simulink model "SistemaCompleto_PMSM"  (R2025a)
settings: Solver=VariableStepAuto  StartTime=0.0  StopTime=3  RelTol=1e-3
PostLoadFcn:
  | parametros_sistema_completo
  | run("parametros_sistema_completo.mlx")
values from neighbouring files (symbols this model uses):
  a_cu = 3.9e-3    (= 0.0039)    [parametros_sistema_completo.m]    (also in workspace_params.mat)
  b_eq = params.b_total    [calcular_matriz_AO.m]    (also in calculo_incertidumbre_y_control.m = b_m + b_l/(r^2); parametros_sistema_completo.m = 2.19444444444e-05; workspace_params.mat = 2.19444444444e-05)
  C_ts = C_ts * (1 + tol_pct)    [calculo_incertidumbre_y_control.m]    (also in parametros_sistema_completo.m = 0.818; workspace_params.mat = 0.818)
  g = 9.80665    [parametros_sistema_completo.m]    (also in workspace_params.mat)
  J_eq = params.J_total    [calcular_matriz_AO.m]    (also in calculo_incertidumbre_y_control.m = J_m + J_l/r^2; parametros_sistema_completo.m = 1.97847222222e-05; workspace_params.mat = 3.28055555556e-05)
  k_l = m*l_cm + m_l*l_l    [calculo_incertidumbre_y_control.m]    (also in parametros_sistema_completo.m = 0.25; workspace_params.mat = 0.625)
  L_d = L_d    * (1 - tol_pct)    [calculo_incertidumbre_y_control.m]    (also in parametros_sistema_completo.m = 0.0066; workspace_params.mat = 0.0066)
  L_ls = L_ls   * (1 - tol_pct)    [calculo_incertidumbre_y_control.m]    (also in parametros_sistema_completo.m = 0.0008; workspace_params.mat = 0.0008)
  L_q = L_q    * (1 - tol_pct)    [calculo_incertidumbre_y_control.m]    (also in parametros_sistema_completo.m = 0.0058; workspace_params.mat = 0.0058)
  lambda_r = lambda_r * (1 + tol_pct)    [calculo_incertidumbre_y_control.m]    (also in parametros_sistema_completo.m = 0.016; workspace_params.mat = 0.016)
  P_p = 3    [parametros_sistema_completo.m]    (also in workspace_params.mat)
  r = params.r_red    [calcular_matriz_AO.m]    (also in parametros_sistema_completo.m = 120; workspace_params.mat = 120)
  R_sREF = R_sREF * (1 - tol_pct)    [calculo_incertidumbre_y_control.m]    (also in parametros_sistema_completo.m = 1.02; workspace_params.mat = 1.02)
  R_ts_amb = R_ts_amb * (1 - tol_pct)    [calculo_incertidumbre_y_control.m]    (also in parametros_sistema_completo.m = 146.7; workspace_params.mat = 146.7)
  T_amb = 20    [parametros_sistema_completo.m]    (also in workspace_params.mat)
  T_sREF = 20    [parametros_sistema_completo.m]    (also in workspace_params.mat)
undefined symbols (not defined in the file or in its folder): i_ds_inicial
libraries: eeStairGenerator x2
settings Model: Creator=Francisco  LastModifiedBy=Francisco
settings DebuggingCC: UnderspecifiedInitializationDetection=Classic  MergeDetectMultiDrivingBlocksExec=none
settings ModelReferenceCC: PropagateSignalLabelsOutOfModel=off
settings RTWCC: GPUComputeCapability=3.5

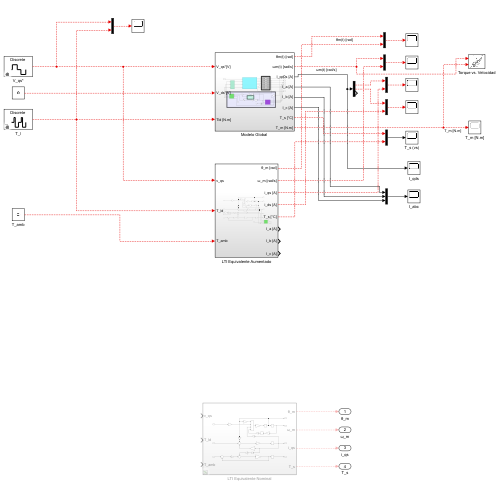
[thumbnail: Simulink's stored preview of the top-level diagram]
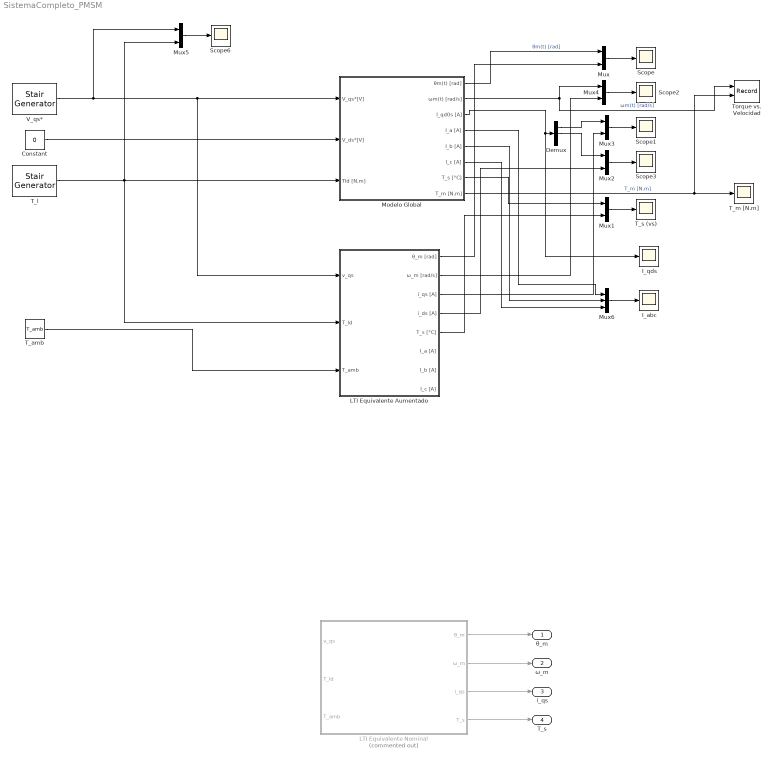
== system SistemaCompleto_PMSM ==
  Constant : Constant  Value=0
  Demux : Demux  Outputs=3
  I_abc : Scope
      settings: ActiveDisplayYMinimum=-11.027390626424687  ActiveDisplayYMaximum=9.9575916434176612  DataLoggingVariableName=ScopeData8
  I_qds : Scope
      settings: ActiveDisplayYMinimum=-9.49860290767503  ActiveDisplayYMaximum=9.6412352540190742  DataLoggingVariableName=ScopeData3
  LTI Equivalente Aumentado : Subsystem
  LTI Equivalente Nominal : Subsystem  Commented=on
  "Modelo Global " : Subsystem
  Mux{,1..5} (6 alike) : Mux  Inputs=2
  Mux6 : Mux  Inputs=3
  Scope{,1..3,6} (5 alike) : Scope
      Scope settings: ActiveDisplayYMinimum=-1  ActiveDisplayYMaximum=1
      Scope1 settings: ActiveDisplayYMinimum=-1  ActiveDisplayYMaximum=1  DataLoggingVariableName=ScopeData2
      Scope2 settings: ActiveDisplayYMinimum=-1  ActiveDisplayYMaximum=1
      Scope3 settings: ActiveDisplayYMinimum=-6.8361156933848816E-13  ActiveDisplayYMaximum=1.2107764476761756E-12  DataLoggingVariableName=ScopeData4
      Scope6 settings: ActiveDisplayYMinimum=-1  ActiveDisplayYMaximum=1  DataLoggingVariableName=ScopeData7
  T_amb : Constant  Value=T_amb
  T_l : eeStairGenerator/Stair Generator  LabelModeActiveChoice=Discrete  TimeInput=[0 0.3 0.5 0.9 1.3 1.5 1.9]  AmplitudeInput=[0 6.28 -6.28 0 6.28 -6.28 0]  SampleTime=0.001  RepeatPattern=off  OutDataTypeStr=double
      settings: LibrarySourceBlock=ee_sl_lib/General Control/Stair Generator
  T_m [N.m] : Scope
      settings: ActiveDisplayYMinimum=-0.86646302297159927  ActiveDisplayYMaximum=1.6077968765433432  DataLoggingVariableName=ScopeData6
  T_s (vs) : Scope
      settings: ActiveDisplayYMinimum=18.3730242701774  ActiveDisplayYMaximum=30.348736241613476  DataLoggingVariableName=ScopeData5
  Torque vs. Velocidad : Record  NumPorts=2.0  FileSettingsInternal="{\"entries\":[{\"content\":{\"excelSettings\":{\"content\":{},\"type\":\"Streamout.ExcelSettings\"},\"parquetSettings\":{\"content\":{},\"type\":\"Streamout.ParquetSettings\"}},\"type\":\"Streamout.FileSettingStorage\",\"uuid\":\"\"}],\"packageUris\":[\"http:\\/\\/schema.mathworks.com\\/mf0\\/streamout_blocks\\/R2020a\"],\"version\":\"1.0\"}"  FrameSettings=[0, 0]  Layout=[1 1]  SignalsInternal="{\"entries\":[{\"content\":{\"signals\":[{\"content\":{\"blockPath\":[],\"dimensions\":[1],\"domain\":\"\",\"lineColor\":\"#a2142f\",\"plots\":[ 1 ],\"port\":1,\"sid\":[\"\"],\"signalID\":1,\"signalName\":\"Modelo Global :2\"},\"type\":\"RecordBlkView.Signal\",\"uuid\":\"\"},{\"content\":{\"blockPath\":[],\"dimensions\":[1],\"domain\":\"\",\"lineColor\":\"#139fff\",\"plots\":[ 1 ],\"port\":2,\"sid\":[\"\"],\"signalID\":2,\"signalName\":\"Modelo Global :8\"},\"type\":\"RecordBlkView.Signal\",\"uuid\":\"\"},{\"content\":{\"blockPath\":[],\"dimensions\":[1],\"domain\":\"\",\"lineColor\":\"#77ac30\",\"lineWidth\":2,\"port\":1,\"sid\":[\"\"],\"signalID\":3},\"type\":\"RecordBlkView.Signal\",\"uuid\":\"\"},{\"content\":{\"blockPath\":[],\"dimensions\":[1],\"domain\":\"\",\"lineColor\":\"#4dbeee\",\"lineWidth\":2,\"port\":1,\"sid\":[\"\"],\"signalID\":4},\"type\":\"RecordBlkView.Signal\",\"uuid\":\"\"},{\"content\":{\"blockPath\":[],\"dimensions\":[1],\"domain\":\"\",\"lineColor\":\"#a2142f\",\"lineWidth\":2,\"port\":1,\"sid\":[\"\"],\"signalID\":5},\"type\":\"RecordBlkView.Signal\",\"uuid\":\"\"},{\"content\":{\"blockPath\":[],\"dimensions\":[1],\"domain\":\"\",\"lineColor\":\"#139fff\",\"lineWidth\":2,\"port\":1,\"sid\":[\"\"],\"signalID\":6},\"type\":\"RecordBlkView.Signal\",\"uuid\":\"\"}]},\"type\":\"RecordBlkView.InputSignals\",\"uuid\":\"\"}],\"packageUris\":[\"http:\\/\\/schema.mathworks.com\\/mf0\\/streamout_blocks\\/R2020a\"],\"version\":\"1.0\"}"  VisualizationBindings="{\"xyplotplugin\":{\"info\":[{\"series\":[{\"bindingParametersList\":[{\"parameter\":\"X-Axis\",\"signalID\":1,\"signalName\":\"Modelo Global :2\"},{\"parameter\":\"Y-Axis\",\"signalID\":2,\"signalName\":\"Modelo Global :8\"}],\"seriesID\":0}],\"subplotID\":1}]}}"  CompatibilityTag=XY
  V_qs* : eeStairGenerator/Stair Generator  LabelModeActiveChoice=Discrete  TimeInput=[0 0.1 0.7 1.1 1.7]  AmplitudeInput=[0 19.596 0 -19.596 0]  SampleTime=0.001  RepeatPattern=off  OutDataTypeStr=double
      settings: LibrarySourceBlock=ee_sl_lib/General Control/Stair Generator
  θ_m : Outport
  ω_m : Outport  Port=2
  i_qs : Outport  Port=3
  T_s : Outport  Port=4
  wires:
  LTI Equivalente Nominal/1(θ_m) -> θ_m/1
  LTI Equivalente Nominal/2(ω_m) -> ω_m/1
  LTI Equivalente Nominal/3(i_qs) -> i_qs/1
  LTI Equivalente Nominal/4(T_s) -> T_s/1
  V_qs*/1 -> Mux5/1, LTI Equivalente Aumentado/1(v_qs), "Modelo Global "/1(V_qs*[V])
  T_l/1 -> Mux5/2, LTI Equivalente Aumentado/2(T_ld), "Modelo Global "/3(Tld [N.m])
  T_amb/1 -> LTI Equivalente Aumentado/3(T_amb)
  Constant/1 -> "Modelo Global "/2(V_ds*[V])
  LTI Equivalente Aumentado/1(θ_m [rad]) -> Mux/2
  Mux/1 -> Scope/1
  "Modelo Global "/1(θm(t) [rad]) -> Mux/1  "θm(t) [rad]"
  "Modelo Global "/3(I_qd0s [A]) -> I_qds/1, Demux/1
  Demux/1 -> Mux3/1
  Demux/2 -> Mux2/1
  LTI Equivalente Aumentado/3(i_qs [A]) -> Mux3/2
  LTI Equivalente Aumentado/4(i_ds [A]) -> Mux2/2
  Mux3/1 -> Scope1/1
  Mux2/1 -> Scope3/1
  "Modelo Global "/7(T_s [°C]) -> Mux1/1
  LTI Equivalente Aumentado/5(T_s [°C]) -> Mux1/2
  Mux1/1 -> T_s (vs)/1
  Mux4/1 -> Scope2/1
  "Modelo Global "/2(ωm(t) [rad/s]) -> Mux4/1, Torque vs. Velocidad/1  "ωm(t) [rad/s]"
  LTI Equivalente Aumentado/2(ω_m [rad/s]) -> Mux4/2
  "Modelo Global "/8(T_m [N.m]) -> T_m [N.m]/1, Torque vs. Velocidad/2  "T_m [N.m]"
  Mux5/1 -> Scope6/1
  Mux6/1 -> I_abc/1
  "Modelo Global "/4(I_a [A]) -> Mux6/1
  "Modelo Global "/5(I_b [A]) -> Mux6/2
  "Modelo Global "/6(I_c [A]) -> Mux6/3

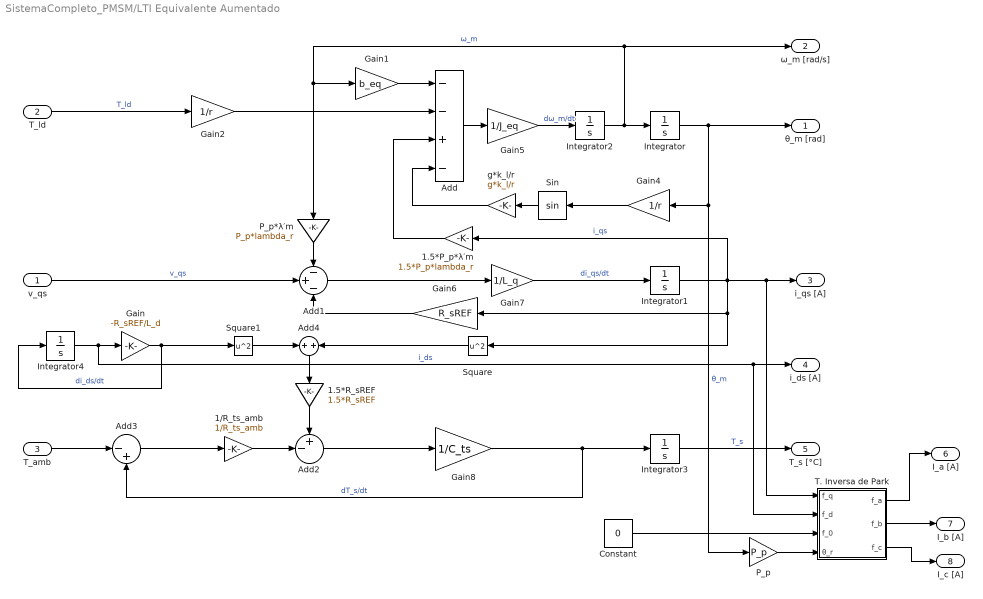
== system SistemaCompleto_PMSM/LTI Equivalente Aumentado ==
  v_qs : Inport
  T_ld : Inport  Port=2
  T_amb : Inport  Port=3
  1.5*P_p*λ′m : Gain  Gain=1.5*P_p*lambda_r
  1.5*R_sREF : Gain  Gain=1.5*R_sREF
  1/R_ts_amb : Gain  Gain=1/R_ts_amb
  Add : Sum  Inputs=--+-
  Add1 : Sum  Inputs=-+-
  Add2 : Sum  Inputs=+-|
  Add3 : Sum  Inputs=|-+
  Add4 : Sum
  Constant : Constant  Value=0
  Gain : Gain  Gain=-R_sREF/L_d
  Gain1 : Gain  Gain=b_eq
  Gain2 : Gain  Gain=1/r
  Gain4 : Gain  Gain=1/r
  Gain5 : Gain  Gain=1/J_eq
  Gain6 : Gain  Gain=R_sREF
  Gain7 : Gain  Gain=1/L_q
  Gain8 : Gain  Gain=1/C_ts
  Integrator{,1..2,4} (4 alike) : Integrator
  Integrator3 : Integrator  InitialCondition=T_amb
  P_p : Gain  Gain=P_p
  P_p*λ′m : Gain  Gain=P_p*lambda_r
  Sin : Trigonometry
  Square : Math  Operator=square
  Square1 : Math  Operator=square
  T. Inversa de Park : Subsystem
  g*k_l/r : Gain  Gain=g*k_l/r
  θ_m [rad] : Outport
  ω_m [rad/s] : Outport  Port=2
  i_qs [A] : Outport  Port=3
  i_ds [A] : Outport  Port=4
  T_s [°C] : Outport  Port=5
  I_a [A] : Outport  Port=6
  I_b [A] : Outport  Port=7
  I_c [A] : Outport  Port=8
  wires:
  P_p*λ′m/1 -> Add1/1
  Add/1 -> Gain5/1
  T_amb/1 -> Add3/1
  g*k_l/r/1 -> Add/4
  Gain1/1 -> Add/1
  v_qs/1 -> Add1/2  "v_qs"
  1.5*P_p*λ′m/1 -> Add/3
  Gain6/1 -> Add1/3
  Gain2/1 -> Add/2
  T_ld/1 -> Gain2/1  "T_ld"
  Sin/1 -> g*k_l/r/1
  1.5*R_sREF/1 -> Add2/1
  1/R_ts_amb/1 -> Add2/2
  Add2/1 -> Gain8/1
  Square/1 -> Add4/2
  Gain5/1 -> Integrator2/1  "dω_m/dt"
  Gain4/1 -> Sin/1
  Add3/1 -> 1/R_ts_amb/1
  Integrator3/1 -> T_s [°C]/1  "T_s"
  Gain7/1 -> Integrator1/1  "di_qs/dt"
  Integrator/1 -> P_p/1, Gain4/1, θ_m [rad]/1  "θ_m"
  Gain8/1 -> Add3/2, Integrator3/1  "dT_s/dt"
  Integrator1/1 -> Square/1, Gain6/1, T. Inversa de Park/1(f_q), i_qs [A]/1, 1.5*P_p*λ′m/1  "i_qs"
  Integrator2/1 -> Integrator/1, P_p*λ′m/1, Gain1/1, ω_m [rad/s]/1  "ω_m"
  Add1/1 -> Gain7/1
  Gain/1 -> Integrator4/1, Square1/1  "di_ds/dt"
  Integrator4/1 -> T. Inversa de Park/2(f_d), i_ds [A]/1, Gain/1  "i_ds"
  Square1/1 -> Add4/1
  Add4/1 -> 1.5*R_sREF/1
  P_p/1 -> T. Inversa de Park/4(θ_r)
  T. Inversa de Park/3(f_c) -> I_c [A]/1
  T. Inversa de Park/2(f_b) -> I_b [A]/1
  T. Inversa de Park/1(f_a) -> I_a [A]/1
  Constant/1 -> T. Inversa de Park/3(f_0)

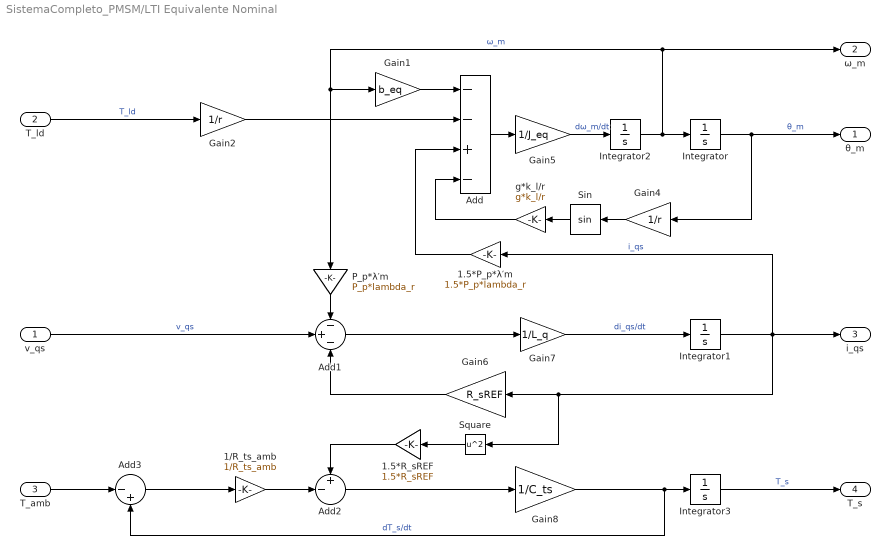
== system SistemaCompleto_PMSM/LTI Equivalente Nominal ==
  v_qs : Inport
  T_ld : Inport  Port=2
  T_amb : Inport  Port=3
  1.5*P_p*λ′m : Gain  Gain=1.5*P_p*lambda_r
  1.5*R_sREF : Gain  Gain=1.5*R_sREF
  1/R_ts_amb : Gain  Gain=1/R_ts_amb
  Add : Sum  Inputs=--+-
  Add1 : Sum  Inputs=-+-
  Add2 : Sum  Inputs=+-|
  Add3 : Sum  Inputs=|-+
  Gain1 : Gain  Gain=b_eq
  Gain2 : Gain  Gain=1/r
  Gain4 : Gain  Gain=1/r
  Gain5 : Gain  Gain=1/J_eq
  Gain6 : Gain  Gain=R_sREF
  Gain7 : Gain  Gain=1/L_q
  Gain8 : Gain  Gain=1/C_ts
  Integrator{,1..3} (4 alike) : Integrator
  P_p*λ′m : Gain  Gain=P_p*lambda_r
  Sin : Trigonometry
  Square : Math  Operator=square
  g*k_l/r : Gain  Gain=g*k_l/r
  θ_m : Outport
  ω_m : Outport  Port=2
  i_qs : Outport  Port=3
  T_s : Outport  Port=4
  wires:
  Add1/1 -> Gain7/1
  Integrator2/1 -> ω_m/1, Gain1/1, P_p*λ′m/1, Integrator/1  "ω_m"
  Integrator1/1 -> i_qs/1, 1.5*P_p*λ′m/1, Square/1, Gain6/1  "i_qs"
  Gain8/1 -> Add3/2, Integrator3/1  "dT_s/dt"
  Integrator/1 -> θ_m/1, Gain4/1  "θ_m"
  Gain7/1 -> Integrator1/1  "di_qs/dt"
  Integrator3/1 -> T_s/1  "T_s"
  Add3/1 -> 1/R_ts_amb/1
  Gain4/1 -> Sin/1
  Gain5/1 -> Integrator2/1  "dω_m/dt"
  Square/1 -> 1.5*R_sREF/1
  Add2/1 -> Gain8/1
  1/R_ts_amb/1 -> Add2/2
  1.5*R_sREF/1 -> Add2/1
  Sin/1 -> g*k_l/r/1
  T_ld/1 -> Gain2/1  "T_ld"
  Gain2/1 -> Add/2
  Gain6/1 -> Add1/3
  1.5*P_p*λ′m/1 -> Add/3
  v_qs/1 -> Add1/2  "v_qs"
  Gain1/1 -> Add/1
  g*k_l/r/1 -> Add/4
  T_amb/1 -> Add3/1
  Add/1 -> Gain5/1
  P_p*λ′m/1 -> Add1/1

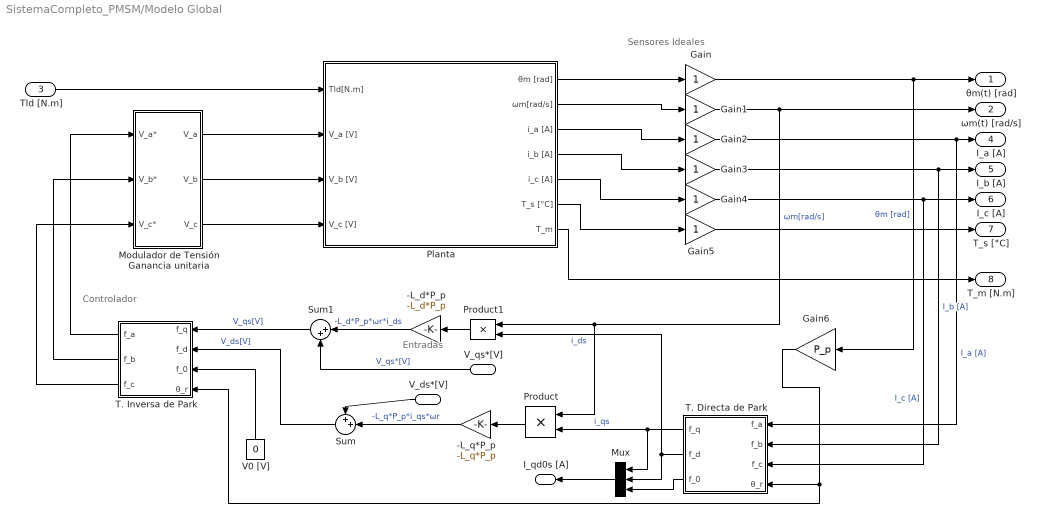
== system SistemaCompleto_PMSM/Modelo Global  ==
  note: Entradas
  note: Sensores Ideales
  note: Controlador
  V_qs*[V] : Inport
  V_ds*[V] : Inport  Port=2
  Tld [N.m] : Inport  Port=3
  -L_d*P_p : Gain  Gain=-L_d*P_p
  -L_q*P_p : Gain  Gain=-L_q*P_p
  Gain{,1..5} (6 alike) : Gain
  Gain6 : Gain  Gain=P_p
  Modulador de Tensión Ganancia unitaria : Subsystem
  Mux : Mux  Inputs=3
  Planta : Subsystem
  Product : Product
  Product1 : Product
  Sum : Sum  Inputs=++|
  Sum1 : Sum  Inputs=|++
  T. Directa de Park : Subsystem
  T. Inversa de Park : Subsystem
  V0 [V] : Constant  Value=0
  θm(t) [rad] : Outport
  ωm(t) [rad/s] : Outport  Port=2
  I_qd0s [A] : Outport  Port=3
  I_a [A] : Outport  Port=4
  I_b [A] : Outport  Port=5
  I_c [A] : Outport  Port=6
  T_s [°C] : Outport  Port=7
  T_m [N.m] : Outport  Port=8
  wires:
  Gain/1 -> Gain6/1, θm(t) [rad]/1  "θm [rad]"
  V0 [V]/1 -> T. Inversa de Park/3(f_0)
  Planta/4(i_b [A]) -> Gain3/1
  Gain4/1 -> T. Directa de Park/3(f_c), I_c [A]/1  "I_c [A]"
  Tld [N.m]/1 -> Planta/1(Tld[N.m])
  Planta/1(θm [rad]) -> Gain/1
  Planta/2(ωm[rad/s]) -> Gain1/1
  Planta/3(i_a [A]) -> Gain2/1
  Planta/5(i_c [A]) -> Gain4/1
  Planta/6(T_s [°C]) -> Gain5/1
  Gain2/1 -> I_a [A]/1, T. Directa de Park/1(f_a)  "I_a [A]"
  Gain5/1 -> T_s [°C]/1
  Gain6/1 -> T. Directa de Park/4(θ_r), T. Inversa de Park/4(θ_r)
  Gain3/1 -> I_b [A]/1, T. Directa de Park/2(f_b)  "I_b [A]"
  Gain1/1 -> ωm(t) [rad/s]/1, Product1/1, Product/1  "ωm[rad/s]"
  T. Directa de Park/1(f_q) -> Product/2, Mux/1  "i_qs"
  Product/1 -> -L_q*P_p/1
  -L_q*P_p/1 -> Sum/2  "-L_q*P_p*i_qs*ωr"
  V_ds*[V]/1 -> Sum/1
  Sum/1 -> T. Inversa de Park/2(f_d)  "V_ds[V]"
  Sum1/1 -> T. Inversa de Park/1(f_q)  "V_qs[V]"
  T. Inversa de Park/1(f_a) -> Modulador de Tensión Ganancia unitaria/1(V_a*)
  T. Inversa de Park/2(f_b) -> Modulador de Tensión Ganancia unitaria/2(V_b*)
  T. Inversa de Park/3(f_c) -> Modulador de Tensión Ganancia unitaria/3(V_c*)
  Modulador de Tensión Ganancia unitaria/1(V_a) -> Planta/2(V_a [V])
  Modulador de Tensión Ganancia unitaria/2(V_b) -> Planta/3(V_b [V])
  Modulador de Tensión Ganancia unitaria/3(V_c) -> Planta/4(V_c [V])
  T. Directa de Park/2(f_d) -> Product1/2, Mux/2  "i_ds"
  Product1/1 -> -L_d*P_p/1
  V_qs*[V]/1 -> Sum1/2  "V_qs*[V]"
  -L_d*P_p/1 -> Sum1/1  "-L_d*P_p*ωr*i_ds"
  T. Directa de Park/3(f_0) -> Mux/3
  Mux/1 -> I_qd0s [A]/1
  Planta/7(T_m) -> T_m [N.m]/1

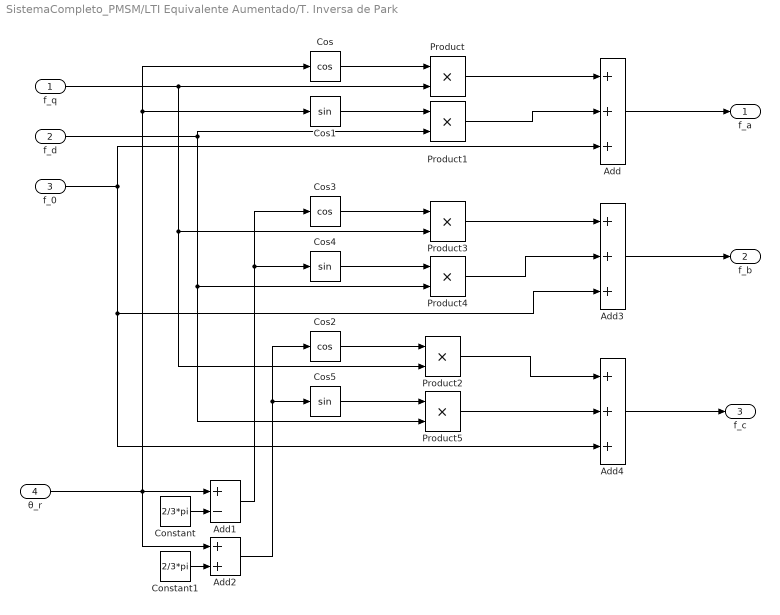
== system SistemaCompleto_PMSM/LTI Equivalente Aumentado/T. Inversa de Park ==
  f_q : Inport
  f_d : Inport  Port=2
  f_0 : Inport  Port=3
  θ_r : Inport  Port=4
  Add : Sum  Inputs=+++
  Add1 : Sum  Inputs=+-
  Add2 : Sum
  Add3 : Sum  Inputs=+++
  Add4 : Sum  Inputs=+++
  Constant : Constant  Value=2/3*pi
  Constant1 : Constant  Value=2/3*pi
  Cos : Trigonometry  Operator=cos
  Cos1 : Trigonometry
  Cos2 : Trigonometry  Operator=cos
  Cos3 : Trigonometry  Operator=cos
  Cos4 : Trigonometry
  Cos5 : Trigonometry
  Product{,1..5} (6 alike) : Product
  f_a : Outport
  f_b : Outport  Port=2
  f_c : Outport  Port=3
  wires:
  Product4/1 -> Add3/2
  Cos1/1 -> Product1/1
  Cos/1 -> Product/1
  Product1/1 -> Add/2
  Add3/1 -> f_b/1
  Cos3/1 -> Product3/1
  Product3/1 -> Add3/1
  f_d/1 -> Product1/2, Product5/2, Product4/2
  Constant1/1 -> Add2/2
  Constant/1 -> Add1/2
  f_0/1 -> Add3/3, Add4/3, Add/3
  Add1/1 -> Cos3/1, Cos4/1
  Product/1 -> Add/1
  f_q/1 -> Product/2, Product2/2, Product3/2
  Cos4/1 -> Product4/1
  θ_r/1 -> Add2/1, Add1/1, Cos/1, Cos1/1
  Add/1 -> f_a/1
  Add4/1 -> f_c/1
  Cos2/1 -> Product2/1
  Cos5/1 -> Product5/1
  Add2/1 -> Cos5/1, Cos2/1
  Product2/1 -> Add4/1
  Product5/1 -> Add4/2

== system SistemaCompleto_PMSM/Modelo Global /Modulador de Tensión Ganancia unitaria ==
  V_a* : Inport
  V_b* : Inport  Port=2
  V_c* : Inport  Port=3
  Gain : Gain
  Gain1 : Gain
  Gain2 : Gain
  V_a : Outport
  V_b : Outport  Port=2
  V_c : Outport  Port=3
  wires:
  V_b*/1 -> Gain/1
  V_a*/1 -> Gain2/1
  V_c*/1 -> Gain1/1
  Gain/1 -> V_b/1
  Gain2/1 -> V_a/1
  Gain1/1 -> V_c/1

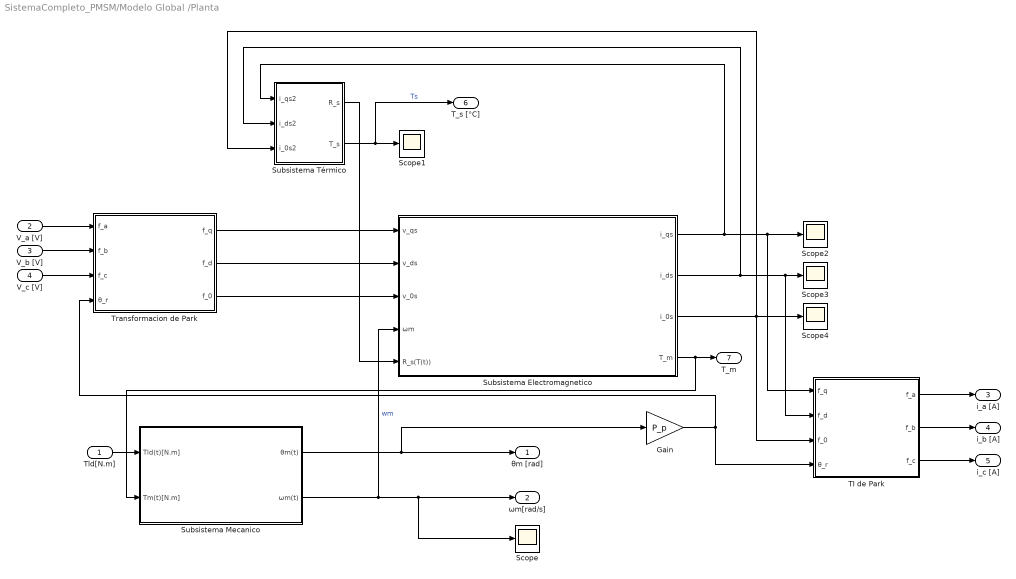
== system SistemaCompleto_PMSM/Modelo Global /Planta ==
  Tld[N.m] : Inport
  V_a [V] : Inport  Port=2
  V_b [V] : Inport  Port=3
  V_c [V] : Inport  Port=4
  Gain : Gain  Gain=P_p
  Scope{,1..4} (5 alike) : Scope
      Scope settings: DataLoggingSaveFormat=Array
      Scope1 settings: DataLoggingSaveFormat=Array
      Scope2 settings: DataLoggingVariableName=ScopeData2  DataLoggingSaveFormat=Array
      Scope3 settings: DataLoggingVariableName=ScopeData3  DataLoggingSaveFormat=Array
      Scope4 settings: DataLoggingVariableName=ScopeData4  DataLoggingSaveFormat=Array
  Subsistema Electromagnetico : Subsystem
  Subsistema Mecanico : Subsystem
  Subsistema Térmico : Subsystem
  TI de Park : Subsystem
  Transformacion de Park : Subsystem
  θm [rad] : Outport
  ωm[rad/s] : Outport  Port=2
  i_a [A] : Outport  Port=3
  i_b [A] : Outport  Port=4
  i_c [A] : Outport  Port=5
  T_s [°C] : Outport  Port=6
  T_m : Outport  Port=7
  wires:
  Subsistema Térmico/1(R_s) -> Subsistema Electromagnetico/5(R_s(T(t)))
  Subsistema Electromagnetico/3(i_0s) -> TI de Park/3(f_0), Scope4/1, Subsistema Térmico/3(i_0s2)
  Subsistema Electromagnetico/4(T_m) -> T_m/1, Subsistema Mecanico/2(Tm(t)[N.m])
  Transformacion de Park/3(f_0) -> Subsistema Electromagnetico/3(v_0s)
  Subsistema Mecanico/2(ωm(t)) -> Subsistema Electromagnetico/4(ωm), Scope/1, ωm[rad/s]/1  "wm"
  Subsistema Electromagnetico/1(i_qs) -> TI de Park/1(f_q), Scope2/1, Subsistema Térmico/1(i_qs2)
  Subsistema Electromagnetico/2(i_ds) -> TI de Park/2(f_d), Scope3/1, Subsistema Térmico/2(i_ds2)
  Transformacion de Park/1(f_q) -> Subsistema Electromagnetico/1(v_qs)
  Subsistema Térmico/2(T_s) -> T_s [°C]/1, Scope1/1  "Ts"
  Transformacion de Park/2(f_d) -> Subsistema Electromagnetico/2(v_ds)
  Subsistema Mecanico/1(θm(t)) -> Gain/1, θm [rad]/1
  Tld[N.m]/1 -> Subsistema Mecanico/1(Tld(t)[N.m])
  Gain/1 -> TI de Park/4(θ_r), Transformacion de Park/4(θ_r)
  TI de Park/1(f_a) -> i_a [A]/1
  TI de Park/2(f_b) -> i_b [A]/1
  TI de Park/3(f_c) -> i_c [A]/1
  V_a [V]/1 -> Transformacion de Park/1(f_a)
  V_b [V]/1 -> Transformacion de Park/2(f_b)
  V_c [V]/1 -> Transformacion de Park/3(f_c)

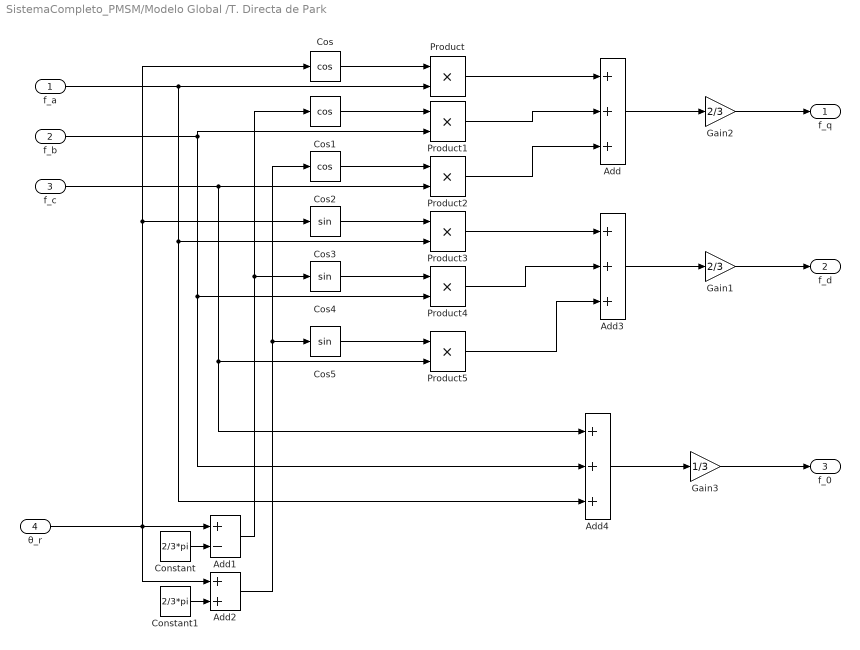
== system SistemaCompleto_PMSM/Modelo Global /T. Directa de Park ==
  f_a : Inport
  f_b : Inport  Port=2
  f_c : Inport  Port=3
  θ_r : Inport  Port=4
  Add : Sum  Inputs=+++
  Add1 : Sum  Inputs=+-
  Add2 : Sum
  Add3 : Sum  Inputs=+++
  Add4 : Sum  Inputs=+++
  Constant : Constant  Value=2/3*pi
  Constant1 : Constant  Value=2/3*pi
  Cos : Trigonometry  Operator=cos
  Cos1 : Trigonometry  Operator=cos
  Cos2 : Trigonometry  Operator=cos
  Cos3 : Trigonometry
  Cos4 : Trigonometry
  Cos5 : Trigonometry
  Gain1 : Gain  Gain=2/3
  Gain2 : Gain  Gain=2/3
  Gain3 : Gain  Gain=1/3
  Product{,1..5} (6 alike) : Product
  f_q : Outport
  f_d : Outport  Port=2
  f_0 : Outport  Port=3
  wires:
  Cos5/1 -> Product5/1
  Gain2/1 -> f_q/1
  Product5/1 -> Add3/3
  Add/1 -> Gain2/1
  θ_r/1 -> Cos3/1, Cos/1, Add1/1, Add2/1
  Cos4/1 -> Product4/1
  Cos2/1 -> Product2/1
  f_a/1 -> Add4/3, Product3/2, Product/2
  Product/1 -> Add/1
  Add1/1 -> Cos1/1, Cos4/1
  f_c/1 -> Product2/2, Product5/2, Add4/1
  Constant/1 -> Add1/2
  Constant1/1 -> Add2/2
  f_b/1 -> Product1/2, Product4/2, Add4/2
  Add2/1 -> Cos2/1, Cos5/1
  Add4/1 -> Gain3/1
  Product3/1 -> Add3/1
  Product2/1 -> Add/3
  Gain3/1 -> f_0/1
  Cos3/1 -> Product3/1
  Add3/1 -> Gain1/1
  Gain1/1 -> f_d/1
  Product1/1 -> Add/2
  Cos/1 -> Product/1
  Cos1/1 -> Product1/1
  Product4/1 -> Add3/2

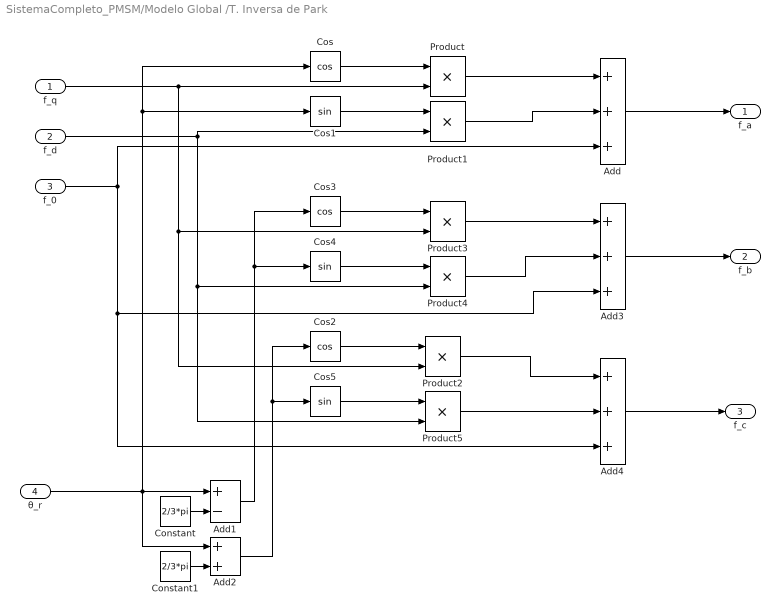
== system SistemaCompleto_PMSM/Modelo Global /T. Inversa de Park ==
  f_q : Inport
  f_d : Inport  Port=2
  f_0 : Inport  Port=3
  θ_r : Inport  Port=4
  Add : Sum  Inputs=+++
  Add1 : Sum  Inputs=+-
  Add2 : Sum
  Add3 : Sum  Inputs=+++
  Add4 : Sum  Inputs=+++
  Constant : Constant  Value=2/3*pi
  Constant1 : Constant  Value=2/3*pi
  Cos : Trigonometry  Operator=cos
  Cos1 : Trigonometry
  Cos2 : Trigonometry  Operator=cos
  Cos3 : Trigonometry  Operator=cos
  Cos4 : Trigonometry
  Cos5 : Trigonometry
  Product{,1..5} (6 alike) : Product
  f_a : Outport
  f_b : Outport  Port=2
  f_c : Outport  Port=3
  wires:
  Product4/1 -> Add3/2
  Cos1/1 -> Product1/1
  Cos/1 -> Product/1
  Product1/1 -> Add/2
  Add3/1 -> f_b/1
  Cos3/1 -> Product3/1
  Product3/1 -> Add3/1
  f_d/1 -> Product1/2, Product5/2, Product4/2
  Constant1/1 -> Add2/2
  Constant/1 -> Add1/2
  f_0/1 -> Add3/3, Add4/3, Add/3
  Add1/1 -> Cos3/1, Cos4/1
  Product/1 -> Add/1
  f_q/1 -> Product/2, Product2/2, Product3/2
  Cos4/1 -> Product4/1
  θ_r/1 -> Add2/1, Add1/1, Cos/1, Cos1/1
  Add/1 -> f_a/1
  Add4/1 -> f_c/1
  Cos2/1 -> Product2/1
  Cos5/1 -> Product5/1
  Add2/1 -> Cos5/1, Cos2/1
  Product2/1 -> Add4/1
  Product5/1 -> Add4/2

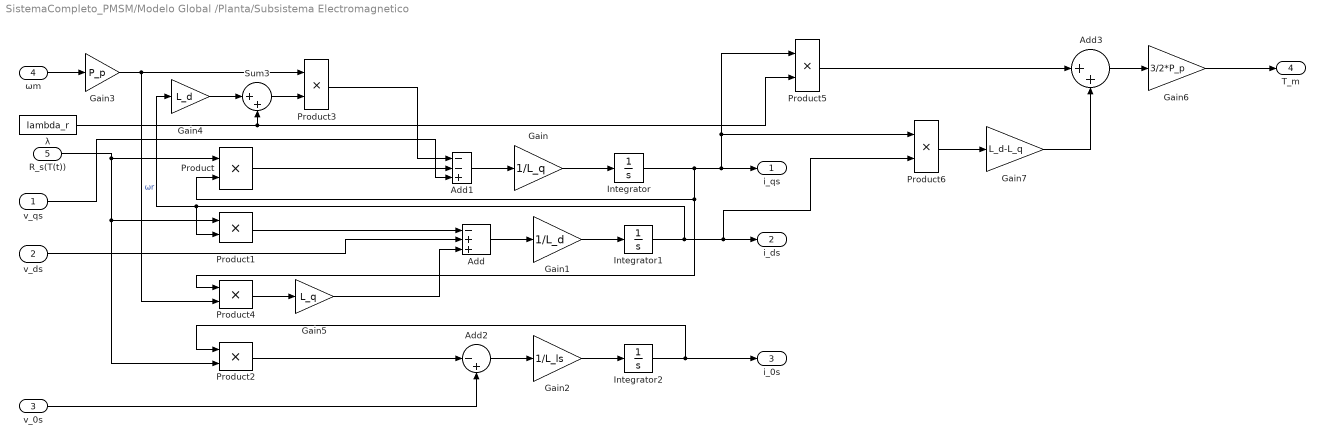
== system SistemaCompleto_PMSM/Modelo Global /Planta/Subsistema Electromagnetico ==
  v_qs : Inport
  v_ds : Inport  Port=2
  v_0s : Inport  Port=3
  ωm : Inport  Port=4
  R_s(T(t)) : Inport  Port=5
  Add : Sum  Inputs=-++
  Add1 : Sum  Inputs=--+
  Add2 : Sum  Inputs=|-+
  Add3 : Sum  Inputs=|++
  Gain : Gain  Gain=1/L_q
  Gain1 : Gain  Gain=1/L_d
  Gain2 : Gain  Gain=1/L_ls
  Gain3 : Gain  Gain=P_p
  Gain4 : Gain  Gain=L_d
  Gain5 : Gain  Gain=L_q
  Gain6 : Gain  Gain=3/2*P_p
  Gain7 : Gain  Gain=L_d-L_q
  Integrator : Integrator
  Integrator1 : Integrator  InitialCondition=i_ds_inicial
  Integrator2 : Integrator
  Product{,1..6} (7 alike) : Product
  Sum3 : Sum  Inputs=|++
  λ : Constant  Value=lambda_r
  i_qs : Outport
  i_ds : Outport  Port=2
  i_0s : Outport  Port=3
  T_m : Outport  Port=4
  wires:
  v_0s/1 -> Add2/2
  Gain5/1 -> Add/3
  Gain3/1 -> Product4/2, Product3/1  "ωr"
  Integrator/1 -> Product4/1, Product/2, i_qs/1, Product5/1, Product6/1
  v_qs/1 -> Add1/3
  R_s(T(t))/1 -> Product2/2, Product1/1, Product/1
  Gain4/1 -> Sum3/1
  Product1/1 -> Add/1
  Integrator2/1 -> i_0s/1, Product2/1
  Sum3/1 -> Product3/2
  Integrator1/1 -> Gain4/1, Product1/2, i_ds/1, Product6/2
  Product/1 -> Add1/2
  Product4/1 -> Gain5/1
  ωm/1 -> Gain3/1
  Add3/1 -> Gain6/1
  Gain/1 -> Integrator/1
  Gain6/1 -> T_m/1
  Product2/1 -> Add2/1
  λ/1 -> Sum3/2, Product5/2
  Gain1/1 -> Integrator1/1
  Add/1 -> Gain1/1
  Add1/1 -> Gain/1
  Product6/1 -> Gain7/1
  Product3/1 -> Add1/1
  Gain2/1 -> Integrator2/1
  Gain7/1 -> Add3/2
  v_ds/1 -> Add/2
  Add2/1 -> Gain2/1
  Product5/1 -> Add3/1

== system SistemaCompleto_PMSM/Modelo Global /Planta/Subsistema Mecanico ==
  Tld(t)[N.m] : Inport
  Tm(t)[N.m] : Inport  Port=2
  1/J_eq[kg.m2] : Gain  Gain=1/J_eq
  Gain : Gain  Gain=1/r
  Gain1 : Gain  Gain=1/r
  Integrator : Integrator
  Integrator1 : Integrator
  Sin : Trigonometry
  Sum : Sum  Inputs=-+-
  Sum1 : Sum
  "[N.m/rad]" : Gain  Gain=g*k_l/r
  b_eq[N.m/rad/s] : Gain  Gain=b_eq
  θm(t) : Outport
  ωm(t) : Outport  Port=2
  wires:
  Gain1/1 -> Sin/1
  Sin/1 -> "[N.m/rad]"/1  "θm[rad]"
  Integrator1/1 -> Integrator/1, ωm(t)/1, b_eq[N.m/rad/s]/1  "ωm[rad/s]"
  Tld(t)[N.m]/1 -> Sum1/1
  b_eq[N.m/rad/s]/1 -> Sum/3
  1/J_eq[kg.m2]/1 -> Integrator1/1  "dω/dt [rad/s^2]"
  Gain/1 -> Sum/1
  "[N.m/rad]"/1 -> Sum1/2
  Integrator/1 -> θm(t)/1, Gain1/1  "θm[rad]"
  Sum/1 -> 1/J_eq[kg.m2]/1
  Tm(t)[N.m]/1 -> Sum/2
  Sum1/1 -> Gain/1

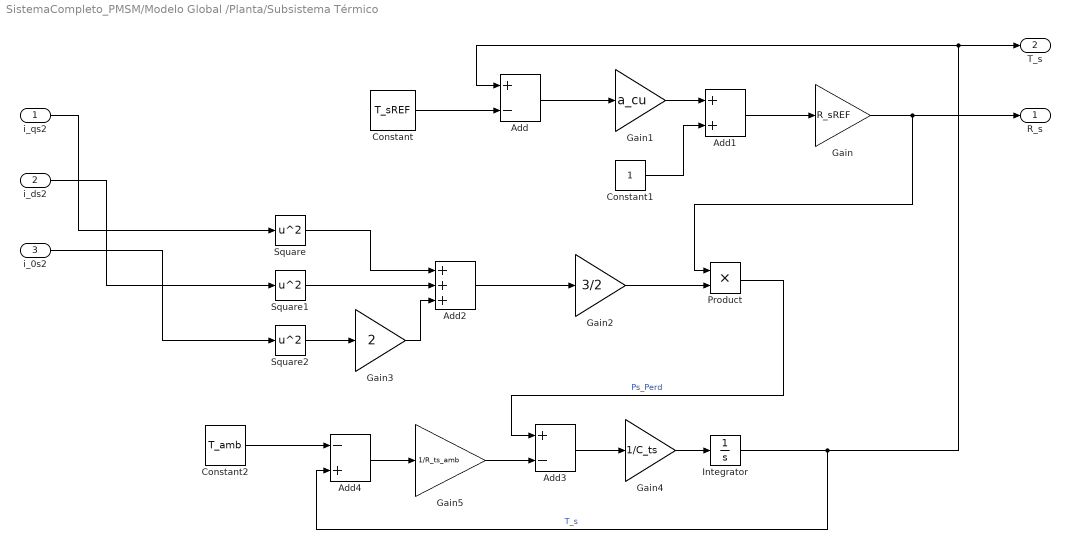
== system SistemaCompleto_PMSM/Modelo Global /Planta/Subsistema Térmico ==
  i_qs2 : Inport
  i_ds2 : Inport  Port=2
  i_0s2 : Inport  Port=3
  Add : Sum  Inputs=+-
  Add1 : Sum
  Add2 : Sum  Inputs=+++
  Add3 : Sum  Inputs=+-
  Add4 : Sum  Inputs=-+
  Constant : Constant  Value=T_sREF
  Constant1 : Constant
  Constant2 : Constant  Value=T_amb
  Gain : Gain  Gain=R_sREF
  Gain1 : Gain  Gain=a_cu
  Gain2 : Gain  Gain=3/2
  Gain3 : Gain  Gain=2
  Gain4 : Gain  Gain=1/C_ts
  Gain5 : Gain  Gain=1/R_ts_amb
  Integrator : Integrator  InitialCondition=20
  Product : Product
  Square : Math  Operator=square  OutDataTypeStr=double
  Square1 : Math  Operator=square
  Square2 : Math  Operator=square
  R_s : Outport
  T_s : Outport  Port=2
  wires:
  Constant1/1 -> Add1/2
  Constant/1 -> Add/2
  i_qs2/1 -> Square/1
  Gain/1 -> R_s/1, Product/1
  Square/1 -> Add2/1
  Add2/1 -> Gain2/1
  Constant2/1 -> Add4/1
  i_ds2/1 -> Square1/1
  Gain5/1 -> Add3/2
  Integrator/1 -> Add4/2, T_s/1, Add/1  "T_s"
  Add1/1 -> Gain/1
  i_0s2/1 -> Square2/1
  Square1/1 -> Add2/2
  Product/1 -> Add3/1  "Ps_Perd"
  Gain2/1 -> Product/2
  Add/1 -> Gain1/1
  Square2/1 -> Gain3/1
  Gain1/1 -> Add1/1
  Add3/1 -> Gain4/1
  Add4/1 -> Gain5/1
  Gain3/1 -> Add2/3
  Gain4/1 -> Integrator/1

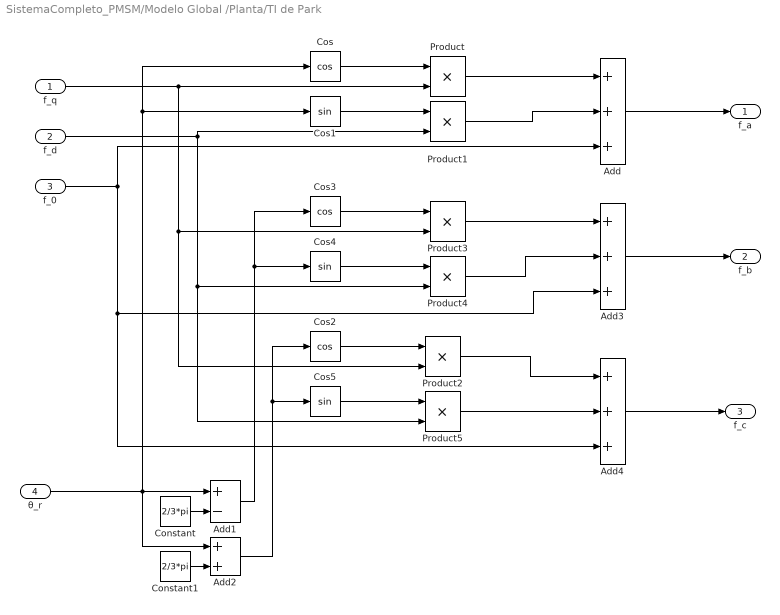
== system SistemaCompleto_PMSM/Modelo Global /Planta/TI de Park ==
  f_q : Inport
  f_d : Inport  Port=2
  f_0 : Inport  Port=3
  θ_r : Inport  Port=4
  Add : Sum  Inputs=+++
  Add1 : Sum  Inputs=+-
  Add2 : Sum
  Add3 : Sum  Inputs=+++
  Add4 : Sum  Inputs=+++
  Constant : Constant  Value=2/3*pi
  Constant1 : Constant  Value=2/3*pi
  Cos : Trigonometry  Operator=cos
  Cos1 : Trigonometry
  Cos2 : Trigonometry  Operator=cos
  Cos3 : Trigonometry  Operator=cos
  Cos4 : Trigonometry
  Cos5 : Trigonometry
  Product{,1..5} (6 alike) : Product
  f_a : Outport
  f_b : Outport  Port=2
  f_c : Outport  Port=3
  wires:
  Product4/1 -> Add3/2
  Cos1/1 -> Product1/1
  Cos/1 -> Product/1
  Product1/1 -> Add/2
  Add3/1 -> f_b/1
  Cos3/1 -> Product3/1
  Product3/1 -> Add3/1
  f_d/1 -> Product1/2, Product5/2, Product4/2
  Constant1/1 -> Add2/2
  Constant/1 -> Add1/2
  f_0/1 -> Add3/3, Add4/3, Add/3
  Add1/1 -> Cos3/1, Cos4/1
  Product/1 -> Add/1
  f_q/1 -> Product/2, Product2/2, Product3/2
  Cos4/1 -> Product4/1
  θ_r/1 -> Add2/1, Add1/1, Cos/1, Cos1/1
  Add/1 -> f_a/1
  Add4/1 -> f_c/1
  Cos2/1 -> Product2/1
  Cos5/1 -> Product5/1
  Add2/1 -> Cos5/1, Cos2/1
  Product2/1 -> Add4/1
  Product5/1 -> Add4/2

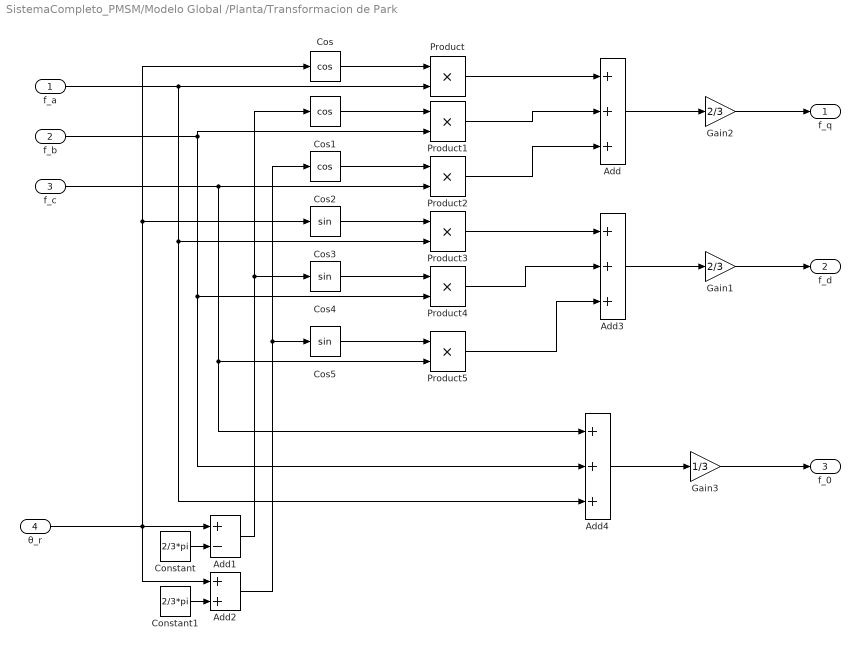
== system SistemaCompleto_PMSM/Modelo Global /Planta/Transformacion de Park ==
  f_a : Inport
  f_b : Inport  Port=2
  f_c : Inport  Port=3
  θ_r : Inport  Port=4
  Add : Sum  Inputs=+++
  Add1 : Sum  Inputs=+-
  Add2 : Sum
  Add3 : Sum  Inputs=+++
  Add4 : Sum  Inputs=+++
  Constant : Constant  Value=2/3*pi
  Constant1 : Constant  Value=2/3*pi
  Cos : Trigonometry  Operator=cos
  Cos1 : Trigonometry  Operator=cos
  Cos2 : Trigonometry  Operator=cos
  Cos3 : Trigonometry
  Cos4 : Trigonometry
  Cos5 : Trigonometry
  Gain1 : Gain  Gain=2/3
  Gain2 : Gain  Gain=2/3
  Gain3 : Gain  Gain=1/3
  Product{,1..5} (6 alike) : Product
  f_q : Outport
  f_d : Outport  Port=2
  f_0 : Outport  Port=3
  wires:
  Cos5/1 -> Product5/1
  Gain2/1 -> f_q/1
  Product5/1 -> Add3/3
  Add/1 -> Gain2/1
  θ_r/1 -> Cos3/1, Cos/1, Add1/1, Add2/1
  Cos4/1 -> Product4/1
  Cos2/1 -> Product2/1
  f_a/1 -> Add4/3, Product3/2, Product/2
  Product/1 -> Add/1
  Add1/1 -> Cos1/1, Cos4/1
  f_c/1 -> Product2/2, Product5/2, Add4/1
  Constant/1 -> Add1/2
  Constant1/1 -> Add2/2
  f_b/1 -> Product1/2, Product4/2, Add4/2
  Add2/1 -> Cos2/1, Cos5/1
  Add4/1 -> Gain3/1
  Product3/1 -> Add3/1
  Product2/1 -> Add/3
  Gain3/1 -> f_0/1
  Cos3/1 -> Product3/1
  Add3/1 -> Gain1/1
  Gain1/1 -> f_d/1
  Product1/1 -> Add/2
  Cos/1 -> Product/1
  Cos1/1 -> Product1/1
  Product4/1 -> Add3/2
